simulink model "ADSBSimulinkExample"  (R2018b)
settings: Solver=FixedStepDiscrete  StartTime=0.0  StopTime=inf  RelTol=1e-3
PreLoadFcn:
  | radioSampleRate = 2.4e6;
  | adsbParam = helperAdsbConfig(radioSampleRate);
  | load dataAdsbBusObjects
  | ReadFromFile = Simulink.Variant('signalSourceNum==1');
  | RTLSDRRadio = Simulink.Variant('signalSourceNum==2');
  | PlutoSDRRadio = Simulink.Variant('signalSourceNum==3');
  | LaunchMap = 0;
  | LogData = 0;
InitFcn:
  | load dataAdsbBusObjects
  | ReadFromFile = Simulink.Variant('signalSourceNum==1');
  | RTLSDRRadio = Simulink.Variant('signalSourceNum==2');
  | PlutoSDRRadio = Simulink.Variant('signalSourceNum==3');
  | helperAdsbCheckModelParams;
undefined symbols (not defined in the file): Fs, ip, usb
libraries: simulink x2, ADSBExampleLib x2, plutoradiolib x1, commsource2 x1, commblksprivate x1, sdrrlib x1
CloseFcn:
  | hFig = findall(0, 'Type', 'figure', 'Tag', 'ADS-B Aircraft Tracking');
  | if ishghandle(hFig)
  | close(hFig);
  | end
  | clear hFig
settings Model: Creator=The MathWorks, Inc.  LastModifiedBy=trevor
settings DataIOCC: LimitDataPoints=on  SaveFormat=Array  SaveOutput=off  SaveTime=off
settings OptimizationCC: BooleanDataType=off  DefaultParameterBehavior=Inlined  LocalBlockOutputs=off  LifeSpan=inf
settings DebuggingCC: AlgebraicLoopMsg=error  SingleTaskRateTransMsg=error  AllowSymbolicDim=off  LibraryContextMissingDiagnostic=none  SFUnexpectedBacktrackingDiag=warning  SFNoUnconditionalDefaultTransitionDiag=warning  SFExecutionAtInitializationDiag=none
settings ModelReferenceCC: PropagateSignalLabelsOutOfModel=off
settings SFSimCC: SimUseLocalCustomCode=off
settings RTWCC: RTWUseLocalCustomCode=off
settings CodeAppCC: StateflowObjectComments=on
settings GRTTargetCC: TargetLangStandard=C89/C90 (ANSI)  GeneratePreprocessorConditionals=Disable all
settings ConfigComp: CovScope=ReferencedModels  CovMetricSettings=dw  CovHtmlReporting=on  CovSaveCumulativeToWorkspaceVar=on  CovSaveSingleToWorkspaceVar=on  CovExternalEMLEnable=off  CovSFcnEnable=off

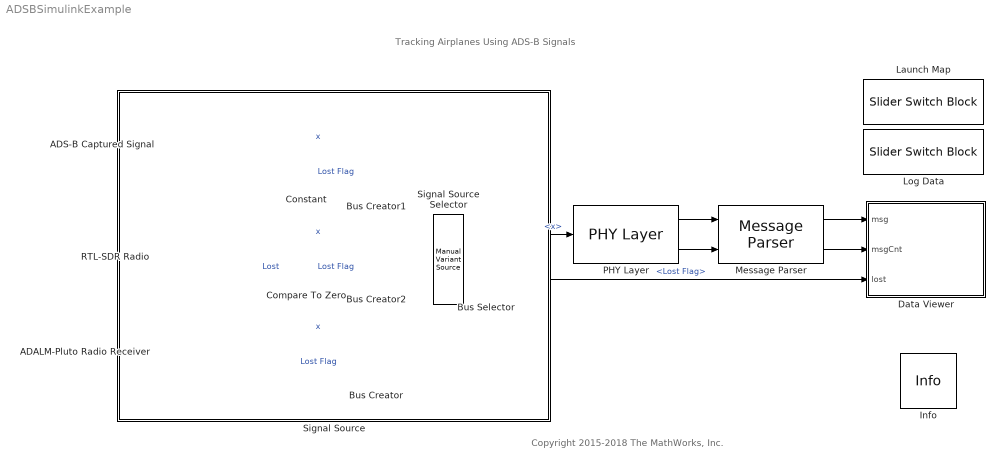
== system ADSBSimulinkExample ==
  note: Tracking Airplanes Using ADS-B Signals
  note: Copyright 2015-2018 The MathWorks, Inc.
  ADALM-Pluto Radio Receiver : plutoradiolib/ADALM-Pluto Radio Receiver  RadioID=usb:0  uri=ip:10.0.0.200  CenterFrequencySource=Dialog  CenterFrequency=1090e6  GainSource=AGC Slow Attack  Gain=10  ChannelMapping=1  BasebandSampleRate=adsbParam.FrontEndSampleRate  OutputDataType=single  SamplesPerFrame=adsbParam.SamplesPerFrame  OverflowOutputPort=on  EnableBurstMode=off  NumFramesInBurst=1  ShowAdvancedProperties=off  UseCustomFilter=off  EnableQuadratureCorrection=on  EnableRFDCCorrection=on  EnableBasebandDCCorrection=on  FrequencyCorrection=0  OverrideSampleTime=off  SampleTime=0.02  DataTimeout=Inf  ENSMPinControlMode=None  BISTLoopbackMode=Disabled  BISTToneInject=Disabled  BISTSignalGen=PRBS  BISTToneFreq=Fs/32  BISTToneLevel=0
      settings: SourceProductName=Communications System Toolbox Support Package for Analog Devices ADALM-Pluto Radio  SourceProductBaseCode=PLUTO
  ADS-B Captured Signal : commsource2/Baseband File Reader  Filename=adsb_capture_01.bb  InheritSampleTimeFromFile=on  SampleTime=1  SamplesPerFrame=adsbParam.SamplesPerFrame  CyclicRepetition=on  FileEndOutputPort=off  SimulateUsing=Code generation
      settings: SourceProductName=Communications Toolbox  SourceProductBaseCode=CM
  Bus Creator : BusCreator  Inputs=2
  Bus Creator1 : BusCreator  Inputs=2
  Bus Creator2 : BusCreator  Inputs=2
  Bus Selector : BusSelector  OutputSignals=x,Lost Flag
  Compare To Zero : simulink/Logic and Bit Operations/Compare To Zero  relop=>  OutDataTypeStr=boolean
  Constant : Constant  Value=0
  Data Viewer : MATLAB Function  StopFcn=|  TreatAsAtomicUnit=on  mask(ADS-B viewer){logfilename=adsb_messages.txt}
      | adsbGUI=findall(0,'type','figure','Tag','ADS-B Aircraft Tracking');
      | if ~isempty(adsbGUI)
      |   viewer=getappdata(adsbGUI,'ViewerHandle');
      |   stop(viewer);
      | end
      mask prompts: logfilename "Log data to file :"
  Info : commblksprivate/Info  SystemSampleTime=-1
      settings: SourceProductName=Communications Toolbox  SourceProductBaseCode=CM
  Launch Map : SliderSwitchBlock  WebBlockId=131
      settings: Values={{'Off', 'On'}, [0 1]}
  Log Data : SliderSwitchBlock  WebBlockId=132
      settings: Values={{'Off', 'On'}, [0 1]}
  Message Parser : ADSBExampleLib/Message Parser  SystemSampleTime=-1
      settings: SourceProductName=Communications Toolbox  SourceProductBaseCode=CM
  PHY Layer : ADSBExampleLib/PHY Layer  SystemSampleTime=-1
      settings: SourceProductName=Communications Toolbox  SourceProductBaseCode=CM
  RTL-SDR Radio : sdrrlib/RTL-SDR Receiver  IPAddress=0  CenterFrequencySource=Dialog  CenterFrequency=1090e6  GainSource=Dialog  Gain=60  ADCRate=adsbParam.FrontEndSampleRate  FrequencyCorrection=0  LostSamplesOutputPort=on  LatencyOutputPort=off  OutputDataType=single  FrameLength=adsbParam.SamplesPerFrame  EnableBurstMode=off  NumFramesInBurst=100  sobjType=sdrr.internal.SDRRTLReceiverSL  dataUDPPort=-1  ctrlUDPPort=-1  subDeviceList=nosubdev  sdrBlockType=SDRBlockTypeSLT.SDRRxBlock  requester=UNUSED_BY_SFCN  sdrExecutionMode=SDRExecutionModeSLT.ExecModeHW  BypassUserLogic=off  DecimatorSelect=DDC decimator  SourceSelect=RF data  SineAmplitude=16000  EnableInternalClock=off  BypassIQBalance=off  IFBandwidth=40e6  ADCRateSource=Dialog  IntermediateFrequency=0  DecimationFactorSource=Dialog  DecimationFactor=512  RFFrequencyIsTunable=logical(0)  SampleTime=(adsbParam.SamplesPerFrame)/(adsbParam.FrontEndSampleRate)  IFBandwidthSource=Dialog  SineFrequency=30000  BypassDCBlockingFilter=off  IntermediateFrequencySource=Dialog  IQBalanceCoefficients=64  SkipAllHardwareResetAndInitialization=off  EnableIQCalibrationTable=on  CacheIQCalibrationTable=off  EnableOffsetTuning=off  EnableRTLAGC=off  EnableTestMode=off  EnableTunerAGC=off  FrequencyCorrectionSource=Dialog  NumMLBuffers=128  NumUSBBuffers=16  RTLCrystalFrequency=28800000  TunerCrystalFrequency=28800000
      settings: SourceProductName=Communications System Toolbox Support Package for RTL-SDR Radio  SourceProductBaseCode=RTLSDR
  Signal Source : Subsystem
      mask Display: disp('')
  Signal Source Selector : simulink/Signal Routing/Manual Variant Source  NumChoices=3  LabelModeActiveChoice=V_2
      settings: SourceProductName=Simulink
  wires:
  Message Parser/1 -> Data Viewer/1(msg)
  Message Parser/2 -> Data Viewer/2(msgCnt)
  PHY Layer/1 -> Message Parser/1
  PHY Layer/2 -> Message Parser/2
  Bus Selector/2 -> Data Viewer/3(lost)  "<Lost Flag>"
  Bus Selector/1 -> PHY Layer/1  "<x>"
  RTL-SDR Radio/1 -> Bus Creator2/1  "x"
  ADS-B Captured Signal/1 -> Bus Creator1/1  "x"
  Bus Creator2/1 -> Signal Source Selector/2
  ADALM-Pluto Radio Receiver/1 -> Bus Creator/1  "x"
  Signal Source Selector/1 -> Bus Selector/1
  Bus Creator/1 -> Signal Source Selector/3
  Bus Creator1/1 -> Signal Source Selector/1
  RTL-SDR Radio/2 -> Compare To Zero/1  "Lost"
  Compare To Zero/1 -> Bus Creator2/2  "Lost Flag"
  Constant/1 -> Bus Creator1/2  "Lost Flag"
  ADALM-Pluto Radio Receiver/2 -> Bus Creator/2  "Lost Flag"

== system ADSBSimulinkExample/Signal Source ==

== matlab function ADSBSimulinkExample/Data Viewer ==
  data: msg input; msgCnt input; lost input; LaunchMap parameter; LogData parameter
function viewer(msg, msgCnt, lost, LaunchMap, LogData)
%#codegen

persistent resetGUI

if isempty(resetGUI)
  resetGUI = true;
end

block = 'ADSBSimulinkExample/Data Viewer';

coder.extrinsic('helperAdsbViewerAdaptor');

coder.extrinsic('get_param','set_param');

Logfilename = get_param(block,'logfilename');

helperAdsbViewerAdaptor(msg, msgCnt, resetGUI, LaunchMap, LogData, Logfilename, lost);

resetGUI = false;
